simulink model "North_Country_Grid_2024a"  (R2024a)
settings: Solver=VariableStepAuto  StartTime=0.0  StopTime=10  RelTol=1e-3
PreLoadFcn:
  | Ts=50e-6;
InitFcn:
  | xInitial = WindFarmType4AverageModelInit;
  | Ts=50e-6;
undefined symbols (not defined in the file or in its folder): D1, D11, Delta, DiscIntNeverNeededParam, find_system, Fnom_I, Fnom_R, Idc_nom, lagging, level, pulse, test_alpha, Vdc_nom, VLL_nom_I, VLL_nom_R
libraries: spsSecondOrderFilterLib x47, powerlib_extras x38, simulink x34, spsThreePhaseVIMeasurementLib x30, spsFirstOrderFilterLib x29, simulink_extras x26, spsabctodq0Lib x25, spsThreePhaseTransformerTwoWindingsLib x19, spsThreePhaseBreakerLib x18, spsThreePhasePISectionLineLib x17, spsControlledVoltageSourceLib x15, spsOnDelayLib x12
(part 5 of 18)

== system North_Country_Grid_2024a/Noble Clinton (Type 4, 100.5 MW)/Wind Farm ==
  note: Turbine and Drive Train
  note: Control
  note: Output
  note: Inverter
      | Average Model
  note: DC-DC Boost Converter
      | Average Model
  "Wind (m/s) " : Inport
  Qref_pu : Inport  Port=2
  -> pu : Gain  Gain=1/(Pnom/(3*sqrt(2)/pi*Vnom_gen))  SaturateOnIntegerOverflow=on  OutDataTypeStr=Inherit: Same as input  ParamDataTypeStr=Inherit: Same as input
  Average Switch Voltage : Subsystem
  B_gen : spsThreePhaseVIMeasurementLib/Three-Phase V-I Measurement  VoltageMeasurement=phase-to-phase  SetLabelV=off  LabelV=Vabc  Vpu=on  VpuLL=off  CurrentMeasurement=yes  SetLabelI=off  LabelI=Iabc  Ipu=on  Pbase=Pnom  Vbase=Vnom_gen  OutputType=Complex  PhasorSimulation=off  PSBequivalent=0
  B_grid : spsThreePhaseVIMeasurementLib/Three-Phase V-I Measurement  VoltageMeasurement=phase-to-ground  SetLabelV=off  LabelV=Vabc  Vpu=on  VpuLL=off  CurrentMeasurement=yes  SetLabelI=off  LabelI=Iabc  Ipu=on  Pbase=Pnom  Vbase=Vnom  OutputType=Complex  PhasorSimulation=off  PSBequivalent=0
  B_grid_conv : spsThreePhaseVIMeasurementLib/Three-Phase V-I Measurement  VoltageMeasurement=phase-to-ground  SetLabelV=off  LabelV=Vabc  Vpu=on  VpuLL=off  CurrentMeasurement=no  SetLabelI=off  LabelI=Iabc  Ipu=on  Pbase=Pnom  Vbase=Vnom  OutputType=Complex  PhasorSimulation=off  PSBequivalent=0
  Bus Creator : BusCreator  Inputs=11
  Bus Selector : BusSelector  OutputSignals="Mechanical.Rotor speed  wm  (pu),Mechanical.Rotor mechanical angle  theta (deg)"
  "Choke " : spsThreePhaseSeriesRLCBranchLib/Three-Phase Series RLC Branch  LConnTagsString=A|B|C  RConnTagsString=A|B|C  BranchType=RL  Resistance=R_RL*Vnom^2/Pnom  Inductance=L_RL*Vnom^2/Pnom/(2*pi*Fnom)  Capacitance=[]  Measurements=None
  Control : Subsystem
  Drive Train : Subsystem  mask(Wind Turbine shaft){H_WT=H_WT, Ksh=Ksh, D_mutual=D_mutual, wbase=2*pi*Fnom/p, w_wt0=w_wt0, torque0=torque0, Ts=Ts}
      mask prompts: H_WT "Wind turbine inertia constant H (s):"; Ksh "Shaft spring constant (pu of nominal mechanical torque/rad):"; D_mutual "Shaft mutual damping (pu of nominal mechanical torque/pu dw):"; wbase "Shaft base speed (rad/s):"; w_wt0 "Turbine initial speed (pu of base speed):"; torque0 "Initial output torque (pu of nominal mechanical torque):"; Ts "Sample time (s):"
      mask help:
      | This block implements a wind turbine drive train model. All shaft parameters are referred to high-speed shaft (generator shaft).
      |
      | The first input is the wind turbine torque in per unit (pu) based on the nominal power of the turbine and the base speed of the generator. The second input is the generator speed in pu based on the base speed of the generator.
      |
      | The outputs are:
      | 1- the transmitted torque of the shaft in pu based on the nominal power of the turbine and the base speed of the generator.
      | 2- the wind turbine speed in pu of the base speed of the generator.
  Filter Q=50 : spsThreePhaseSeriesRLCLoadLib/Three-Phase Series RLC Load  LConnTagsString=A|B|C  Configuration=Y (grounded)  NominalVoltage=Vnom  Vabc=[1e3 1e3 1e3]  Vabcp=[1e3 1e3 1e3]  NominalFrequency=Fnom  UnbalancedPower=off  ActivePower=C_var_filter/Q_filter  InductivePower=0  CapacitivePower=C_var_filter  Pabc=[10e3 9e3 11e3]  QLabc=[100 90 110]  QCabc=[100 90 110]  Pabcp=[10e3 9e3 11e3]  QLabcp=[100 90 110]  QCabcp=[100 90 110]  Measurements=None  LoadType=constant Z
  IL : spsCurrentMeasurementLib/Current Measurement  PhasorSimulation=off  OutputType=Complex  PSBequivalent=0
  Inverter and DC-DC Converter Average Models : Subsystem
  Power base for the Generator : Gain  Gain=Pmec/Pnom  SaturateOnIntegerOverflow=on  OutDataTypeStr=Inherit: Same as input  ParamDataTypeStr=Inherit: Same as input
  Product : Product  RndMeth=Zero
  Series RLC Branch1 : spsSeriesRLCBranchLib/Series RLC Branch  LConnTagsString=__new0  RConnTagsString=__new0  BranchType=RL  Resistance=R_Boost  Inductance=L_Boost  SetiL0=off  InitialCurrent=0  Capacitance=1.0  Setx0=off  InitialVoltage=0  Measurements=Branch current
  Synchronous Machine pu Standard : spsSynchronousMachinepuStandardLib/Synchronous Machine pu Standard  PresetModel=No  MechanicalLoad=Mechanical power Pm  ShowDetailedParameters=on  RotorType=Salient-pole  Units=per unit standard parameters  MeasurementBus=off  NominalParameters="[ Pnom  Vnom_gen Fnom ]"  Reactances1=[ 1.81, 0.3, 0.23, 1.76, 0.65, 0.25, 0.15 ]  Reactances2="[ Xd, Xd1, Xd2, Xq,  Xq2,  Xl ]"  dAxisTimeConstants=Open-circuit  qAxisTimeConstants=Short-circuit  TimeConstants1="[ 4.4849  0.0681  0.1  ]"  TimeConstants2=[ 8.0, 0.03, 1.0, 0.07 ]  TimeConstants3="[  Tdo1  Tdo2  Tq2  ]"  TimeConstants4=[ 8.0, 0.03, 0.3371, 0.0295 ]  TimeConstants5=[ 1.01, 0.053, 0.1 ]  TimeConstants6=[ 1.3201, 0.023, 1.0, 0.07 ]  TimeConstants7="[  1.01  0.053  0.051266  ]"  TimeConstants8=[ 1.3201, 0.0231, 0.3371, 0.0295 ]  StatorResistance=Resistance  Mechanical=[ H F p]  PolePairs=1  InitialConditions=init  SetSaturation=off  Saturation=[0.6404,0.7127,0.8441,0.9214,0.9956,1.082,1.19,1.316,1.457;0.7,0.7698,0.8872,0.9466,0.9969,1.046,1.1,1.151,1.201]  LoadFlowParameters=[1,0,0,0,0]  TsPowergui=0  TsBlock=-1  IterativeModel=Trapezoidal non iterative  IterativeDiscreteModel=Trapezoidal non iterative  BusType=PV  Pref=0  Qref=0  Qmin=-inf  Qmax=inf  PLF=0  QLF=0
  Universal Bridge : spsUniversalBridgeLib/Universal Bridge  Arms=3  SnubberResistance=2*Ts_snub/(Pnom/(1000*2*pi*Fnom*Vnom_gen^2))  SnubberCapacitance=Pnom/(1000*2*pi*Fnom*Vnom_gen^2)  Device=Diodes  Ron=1e-6/Nb_wt  Lon=0  ForwardVoltages="[  0  0  ]"  ForwardVoltage=0  GTOparameters=[ 10e-6 , 20e-6 ]  IGBTparameters=[ 1e-6 , 2e-6 ]  Measurements=None  Measurements_2=None  converterType=Rectifier
  V_ab : spsControlledVoltageSourceLib/Controlled Voltage Source  Initialize=on  Source_Type=AC  Amplitude=0  Phase=0  Frequency=0  Measurements=None
  V_bc : spsControlledVoltageSourceLib/Controlled Voltage Source  Initialize=on  Source_Type=AC  Amplitude=0  Phase=0  Frequency=0  Measurements=None
  Wind Turbine : Subsystem  mask(Wind Turbine){Prated=Pmec, c1_c8=c1_c8, K1_K2=K1_K2, wind0=wind0, Ts=Ts}
      mask prompts: Prated "Nominal mechanical output power (W):"; c1_c8 "Coefficients [c1 ... c8]"; K1_K2 "Parameters [K1 K2]"; wind0 "Initial wind speed (m/s):"; Ts "Sample time (s):"
      mask help:
      | This block implements a generic wind turbine models.
      |
      | The first input is the turbine speed in per unit of the generator base speed. For a synchronous or asynchronous generator, the base speed is the synchronous speed. For a permanent-magnet generator, the base speed is defined as the speed producing nominal voltage at  no load. The second input is the blade pitch angle in degrees. The third input is the wind speed in m/s.
      |
      | The output is the torque applied to the drive train in per unit based on the nominal power of the turbine and the base speed of the generator.
      mask init:
      | c1 = c1_c8(1);
      | c2 = c1_c8(2);
      | c3 = c1_c8(3);
      | c4 = c1_c8(4);
      | c5 = c1_c8(5);
      | c6 = c1_c8(6);
      | c7 = c1_c8(7);;
      | c8 = c1_c8(8);
      | 
      | K1=K1_K2(1);
      | K2=K1_K2(2);
      settings: OpenFcn=power_openblockproxy();
      mask Display: disp('');
  deg->rd : Gain  Gain=pi/180  SaturateOnIntegerOverflow=on  OutDataTypeStr=Inherit: Same as input  ParamDataTypeStr=Inherit: Same as input
  A : PMIOPort  Tag=PMCPort  Side=Left
  B : PMIOPort  Tag=PMCPort  Port=2  Side=Left
  C : PMIOPort  Tag=PMCPort  Port=3  Side=Left
  m : Outport  VectorParamsAs1DForOutWhenUnconnected=off
  wires:
  Wind Turbine/1(Tt (pu)) -> Drive Train/1(T_wt (pu))
  [wr] -> Drive Train/2(Generator speed (pu))
  Drive Train/2(T_shaft (pu)) -> Power base for the Generator/1
  Power base for the Generator/1 -> [Tm]
  "Wind (m/s) "/1 -> Wind Turbine/3(Wind speed (m/s))
  Drive Train/1(W_wt (pu)) -> Wind Turbine/1(W_wt (pu))
  [Pitch] -> Wind Turbine/2(Pitch angle (deg))
  Bus Selector/2 -> deg->rd/1  "<Rotor mechanical angle  theta (deg)>"
  deg->rd/1 -> [angle_rotor]
  Bus Selector/1 -> [wr]  "<Rotor speed  wm  (pu)>"
  [wr] -> Product/1
  Synchronous Machine pu Standard/1 -> Bus Selector/1
  B_grid_conv/1 -> [Vabc_grid_conv]
  [Vabc_LL_stator] -> Bus Creator/1  "Vabc_stator_pu"
  [Iabc_stator] -> Bus Creator/2  "Iabc_stator_pu"
  [Vabc_grid] -> Bus Creator/3  "Vabc_grid_pu"
  Bus Creator/1 -> m/1
  [Vabc_grid_conv] -> Bus Creator/4  "Vabc_grid_conv_pu"
  [Iabc_grid_conv] -> Bus Creator/5  "Iabc_grid_conv_pu"
  [Vf] -> Bus Creator/6  "Vfield_pu"
  [wr] -> Bus Creator/7  "wr_pu"
  [Pm_gen] -> Bus Creator/8  "Pm_gen_pu"
  [Pitch] -> Bus Creator/9  "Pitch_deg"
  [Vdc] -> Bus Creator/10  "Vdc_V"
  [Tm] -> Product/2
  Product/1 -> Synchronous Machine pu Standard/1, [Pm_gen]
  [Iabc_grid_conv] -> Inverter and DC-DC Converter Average Models/2(Iabc_grid_conv)
  Inverter and DC-DC Converter Average Models/3(Vswitch (V)) -> Average Switch Voltage/1(Vswitch)
  IL/1 -> -> pu/1
  [IL] -> Inverter and DC-DC Converter Average Models/1(IL)
  B_grid/1 -> [Vabc_grid]
  B_grid/2 -> [Iabc_grid_conv]
  B_gen/1 -> [Vabc_LL_stator]
  B_gen/2 -> [Iabc_stator]
  [Vabc_grid] -> Control/1(Vabc_grid)
  [Iabc_grid_conv] -> Control/2(Iabc_grid_conv)
  [Vabc_LL_stator] -> Control/3(Vabc_LL_stator)
  [Iabc_stator] -> Control/4(Iabc_stator)
  [Vdc] -> Control/6(Vdc)
  Qref_pu/1 -> Control/7(Qref)
  [angle_rotor] -> Control/8(angle_rotor)
  [wr] -> Control/9(wr)
  Control/1(Uctrl_inverter) -> Inverter and DC-DC Converter Average Models/3(Uctrl_inverter)
  Control/2(Duty_Cycle) -> Inverter and DC-DC Converter Average Models/4(Duty_Cycle)  "Duty_cycle"
  Control/3(Pitch_angle) -> [Pitch]
  Control/4(Vf) -> [Vf]
  Inverter and DC-DC Converter Average Models/4(Vdc (V)) -> [Vdc]
  [Vf] -> Synchronous Machine pu Standard/2
  Inverter and DC-DC Converter Average Models/1(Vab (V)) -> V_ab/1
  Inverter and DC-DC Converter Average Models/2(Vbc (V)) -> V_bc/1
  Control/5(PQ_pu) -> [PQ_pu]
  [PQ_pu] -> Bus Creator/11  "PQ_pu"
  [IL] -> Control/5(IL)
  -> pu/1 -> [IL]
  connections:
  B_gen/RConn1 -- Synchronous Machine pu Standard/RConn1
  B_gen/RConn2 -- Synchronous Machine pu Standard/RConn2
  B_gen/RConn3 -- Synchronous Machine pu Standard/RConn3
  B_grid/RConn1 -- "Choke "/LConn1
  B_grid/RConn2 -- "Choke "/LConn2
  B_grid/RConn3 -- "Choke "/LConn3
  B_grid/LConn1 -- A/RConn1 -- Filter Q=50/LConn1
  B/RConn1 -- B_grid/LConn2 -- Filter Q=50/LConn2
  C/RConn1 -- B_grid/LConn3 -- Filter Q=50/LConn3
  "Choke "/RConn1 -- B_grid_conv/LConn1
  "Choke "/RConn2 -- B_grid_conv/LConn2
  "Choke "/RConn3 -- B_grid_conv/LConn3
  Series RLC Branch1/LConn1 -- Universal Bridge/RConn1
  Average Switch Voltage/LConn1 -- Universal Bridge/RConn2
  V_ab/RConn1 -- B_grid_conv/RConn1
  B_grid_conv/RConn3 -- V_bc/LConn1
  V_bc/RConn1 -- V_ab/LConn1 -- B_grid_conv/RConn2
  Universal Bridge/LConn1 -- B_gen/LConn1
  Universal Bridge/LConn2 -- B_gen/LConn2
  Universal Bridge/LConn3 -- B_gen/LConn3
  Series RLC Branch1/RConn1 -- IL/LConn1
  Average Switch Voltage/RConn1 -- IL/RConn1

== system North_Country_Grid_2024a/Noble Ellenburg (Type 4, 81 MW)/Wind Farm ==
  note: Turbine and Drive Train
  note: Control
  note: Output
  note: Inverter
      | Average Model
  note: DC-DC Boost Converter
      | Average Model
  "Wind (m/s) " : Inport
  Qref_pu : Inport  Port=2
  -> pu : Gain  Gain=1/(Pnom/(3*sqrt(2)/pi*Vnom_gen))  SaturateOnIntegerOverflow=on  OutDataTypeStr=Inherit: Same as input  ParamDataTypeStr=Inherit: Same as input
  Average Switch Voltage : Subsystem
  B_gen : spsThreePhaseVIMeasurementLib/Three-Phase V-I Measurement  VoltageMeasurement=phase-to-phase  SetLabelV=off  LabelV=Vabc  Vpu=on  VpuLL=off  CurrentMeasurement=yes  SetLabelI=off  LabelI=Iabc  Ipu=on  Pbase=Pnom  Vbase=Vnom_gen  OutputType=Complex  PhasorSimulation=off  PSBequivalent=0
  B_grid : spsThreePhaseVIMeasurementLib/Three-Phase V-I Measurement  VoltageMeasurement=phase-to-ground  SetLabelV=off  LabelV=Vabc  Vpu=on  VpuLL=off  CurrentMeasurement=yes  SetLabelI=off  LabelI=Iabc  Ipu=on  Pbase=Pnom  Vbase=Vnom  OutputType=Complex  PhasorSimulation=off  PSBequivalent=0
  B_grid_conv : spsThreePhaseVIMeasurementLib/Three-Phase V-I Measurement  VoltageMeasurement=phase-to-ground  SetLabelV=off  LabelV=Vabc  Vpu=on  VpuLL=off  CurrentMeasurement=no  SetLabelI=off  LabelI=Iabc  Ipu=on  Pbase=Pnom  Vbase=Vnom  OutputType=Complex  PhasorSimulation=off  PSBequivalent=0
  Bus Creator : BusCreator  Inputs=11
  Bus Selector : BusSelector  OutputSignals="Mechanical.Rotor speed  wm  (pu),Mechanical.Rotor mechanical angle  theta (deg)"
  "Choke " : spsThreePhaseSeriesRLCBranchLib/Three-Phase Series RLC Branch  LConnTagsString=A|B|C  RConnTagsString=A|B|C  BranchType=RL  Resistance=R_RL*Vnom^2/Pnom  Inductance=L_RL*Vnom^2/Pnom/(2*pi*Fnom)  Capacitance=[]  Measurements=None
  Control : Subsystem
  Drive Train : Subsystem  mask(Wind Turbine shaft){H_WT=H_WT, Ksh=Ksh, D_mutual=D_mutual, wbase=2*pi*Fnom/p, w_wt0=w_wt0, torque0=torque0, Ts=Ts}
      mask prompts: H_WT "Wind turbine inertia constant H (s):"; Ksh "Shaft spring constant (pu of nominal mechanical torque/rad):"; D_mutual "Shaft mutual damping (pu of nominal mechanical torque/pu dw):"; wbase "Shaft base speed (rad/s):"; w_wt0 "Turbine initial speed (pu of base speed):"; torque0 "Initial output torque (pu of nominal mechanical torque):"; Ts "Sample time (s):"
      mask help:
      | This block implements a wind turbine drive train model. All shaft parameters are referred to high-speed shaft (generator shaft).
      |
      | The first input is the wind turbine torque in per unit (pu) based on the nominal power of the turbine and the base speed of the generator. The second input is the generator speed in pu based on the base speed of the generator.
      |
      | The outputs are:
      | 1- the transmitted torque of the shaft in pu based on the nominal power of the turbine and the base speed of the generator.
      | 2- the wind turbine speed in pu of the base speed of the generator.
  Filter Q=50 : spsThreePhaseSeriesRLCLoadLib/Three-Phase Series RLC Load  LConnTagsString=A|B|C  Configuration=Y (grounded)  NominalVoltage=Vnom  Vabc=[1e3 1e3 1e3]  Vabcp=[1e3 1e3 1e3]  NominalFrequency=Fnom  UnbalancedPower=off  ActivePower=C_var_filter/Q_filter  InductivePower=0  CapacitivePower=C_var_filter  Pabc=[10e3 9e3 11e3]  QLabc=[100 90 110]  QCabc=[100 90 110]  Pabcp=[10e3 9e3 11e3]  QLabcp=[100 90 110]  QCabcp=[100 90 110]  Measurements=None  LoadType=constant Z
  IL : spsCurrentMeasurementLib/Current Measurement  PhasorSimulation=off  OutputType=Complex  PSBequivalent=0
  Inverter and DC-DC Converter Average Models : Subsystem
  Power base for the Generator : Gain  Gain=Pmec/Pnom  SaturateOnIntegerOverflow=on  OutDataTypeStr=Inherit: Same as input  ParamDataTypeStr=Inherit: Same as input
  Product : Product  RndMeth=Zero
  Series RLC Branch1 : spsSeriesRLCBranchLib/Series RLC Branch  LConnTagsString=__new0  RConnTagsString=__new0  BranchType=RL  Resistance=R_Boost  Inductance=L_Boost  SetiL0=off  InitialCurrent=0  Capacitance=1.0  Setx0=off  InitialVoltage=0  Measurements=Branch current
  Synchronous Machine pu Standard : spsSynchronousMachinepuStandardLib/Synchronous Machine pu Standard  PresetModel=No  MechanicalLoad=Mechanical power Pm  ShowDetailedParameters=on  RotorType=Salient-pole  Units=per unit standard parameters  MeasurementBus=off  NominalParameters="[ Pnom  Vnom_gen Fnom ]"  Reactances1=[ 1.81, 0.3, 0.23, 1.76, 0.65, 0.25, 0.15 ]  Reactances2="[ Xd, Xd1, Xd2, Xq,  Xq2,  Xl ]"  dAxisTimeConstants=Open-circuit  qAxisTimeConstants=Short-circuit  TimeConstants1="[ 4.4849  0.0681  0.1  ]"  TimeConstants2=[ 8.0, 0.03, 1.0, 0.07 ]  TimeConstants3="[  Tdo1  Tdo2  Tq2  ]"  TimeConstants4=[ 8.0, 0.03, 0.3371, 0.0295 ]  TimeConstants5=[ 1.01, 0.053, 0.1 ]  TimeConstants6=[ 1.3201, 0.023, 1.0, 0.07 ]  TimeConstants7="[  1.01  0.053  0.051266  ]"  TimeConstants8=[ 1.3201, 0.0231, 0.3371, 0.0295 ]  StatorResistance=Resistance  Mechanical=[ H F p]  PolePairs=1  InitialConditions=init  SetSaturation=off  Saturation=[0.6404,0.7127,0.8441,0.9214,0.9956,1.082,1.19,1.316,1.457;0.7,0.7698,0.8872,0.9466,0.9969,1.046,1.1,1.151,1.201]  LoadFlowParameters=[1 0 0 0 0]  TsPowergui=0  TsBlock=-1  IterativeModel=Trapezoidal non iterative  IterativeDiscreteModel=Trapezoidal non iterative  BusType=PV  Pref=0  Qref=0  Qmin=-inf  Qmax=inf  PLF=0  QLF=0
  Universal Bridge : spsUniversalBridgeLib/Universal Bridge  Arms=3  SnubberResistance=2*Ts_snub/(Pnom/(1000*2*pi*Fnom*Vnom_gen^2))  SnubberCapacitance=Pnom/(1000*2*pi*Fnom*Vnom_gen^2)  Device=Diodes  Ron=1e-6/Nb_wt  Lon=0  ForwardVoltages="[  0  0  ]"  ForwardVoltage=0  GTOparameters=[ 10e-6 , 20e-6 ]  IGBTparameters=[ 1e-6 , 2e-6 ]  Measurements=None  Measurements_2=None  converterType=Rectifier
  V_ab : spsControlledVoltageSourceLib/Controlled Voltage Source  Initialize=on  Source_Type=AC  Amplitude=0  Phase=0  Frequency=0  Measurements=None
  V_bc : spsControlledVoltageSourceLib/Controlled Voltage Source  Initialize=on  Source_Type=AC  Amplitude=0  Phase=0  Frequency=0  Measurements=None
  Wind Turbine : Subsystem  mask(Wind Turbine){Prated=Pmec, c1_c8=c1_c8, K1_K2=K1_K2, wind0=wind0, Ts=Ts}
      mask prompts: Prated "Nominal mechanical output power (W):"; c1_c8 "Coefficients [c1 ... c8]"; K1_K2 "Parameters [K1 K2]"; wind0 "Initial wind speed (m/s):"; Ts "Sample time (s):"
      mask help:
      | This block implements a generic wind turbine models.
      |
      | The first input is the turbine speed in per unit of the generator base speed. For a synchronous or asynchronous generator, the base speed is the synchronous speed. For a permanent-magnet generator, the base speed is defined as the speed producing nominal voltage at  no load. The second input is the blade pitch angle in degrees. The third input is the wind speed in m/s.
      |
      | The output is the torque applied to the drive train in per unit based on the nominal power of the turbine and the base speed of the generator.
      mask init:
      | c1 = c1_c8(1);
      | c2 = c1_c8(2);
      | c3 = c1_c8(3);
      | c4 = c1_c8(4);
      | c5 = c1_c8(5);
      | c6 = c1_c8(6);
      | c7 = c1_c8(7);;
      | c8 = c1_c8(8);
      | 
      | K1=K1_K2(1);
      | K2=K1_K2(2);
      settings: OpenFcn=power_openblockproxy();
      mask Display: disp('');
  deg->rd : Gain  Gain=pi/180  SaturateOnIntegerOverflow=on  OutDataTypeStr=Inherit: Same as input  ParamDataTypeStr=Inherit: Same as input
  A : PMIOPort  Tag=PMCPort  Side=Left
  B : PMIOPort  Tag=PMCPort  Port=2  Side=Left
  C : PMIOPort  Tag=PMCPort  Port=3  Side=Left
  m : Outport  VectorParamsAs1DForOutWhenUnconnected=off
  wires:
  Wind Turbine/1(Tt (pu)) -> Drive Train/1(T_wt (pu))
  [wr] -> Drive Train/2(Generator speed (pu))
  Drive Train/2(T_shaft (pu)) -> Power base for the Generator/1
  Power base for the Generator/1 -> [Tm]
  "Wind (m/s) "/1 -> Wind Turbine/3(Wind speed (m/s))
  Drive Train/1(W_wt (pu)) -> Wind Turbine/1(W_wt (pu))
  [Pitch] -> Wind Turbine/2(Pitch angle (deg))
  Bus Selector/2 -> deg->rd/1  "<Rotor mechanical angle  theta (deg)>"
  deg->rd/1 -> [angle_rotor]
  Bus Selector/1 -> [wr]  "<Rotor speed  wm  (pu)>"
  [wr] -> Product/1
  Synchronous Machine pu Standard/1 -> Bus Selector/1
  B_grid_conv/1 -> [Vabc_grid_conv]
  [Vabc_LL_stator] -> Bus Creator/1  "Vabc_stator_pu"
  [Iabc_stator] -> Bus Creator/2  "Iabc_stator_pu"
  [Vabc_grid] -> Bus Creator/3  "Vabc_grid_pu"
  Bus Creator/1 -> m/1
  [Vabc_grid_conv] -> Bus Creator/4  "Vabc_grid_conv_pu"
  [Iabc_grid_conv] -> Bus Creator/5  "Iabc_grid_conv_pu"
  [Vf] -> Bus Creator/6  "Vfield_pu"
  [wr] -> Bus Creator/7  "wr_pu"
  [Pm_gen] -> Bus Creator/8  "Pm_gen_pu"
  [Pitch] -> Bus Creator/9  "Pitch_deg"
  [Vdc] -> Bus Creator/10  "Vdc_V"
  [Tm] -> Product/2
  Product/1 -> Synchronous Machine pu Standard/1, [Pm_gen]
  [Iabc_grid_conv] -> Inverter and DC-DC Converter Average Models/2(Iabc_grid_conv)
  Inverter and DC-DC Converter Average Models/3(Vswitch (V)) -> Average Switch Voltage/1(Vswitch)
  IL/1 -> -> pu/1
  [IL] -> Inverter and DC-DC Converter Average Models/1(IL)
  B_grid/1 -> [Vabc_grid]
  B_grid/2 -> [Iabc_grid_conv]
  B_gen/1 -> [Vabc_LL_stator]
  B_gen/2 -> [Iabc_stator]
  [Vabc_grid] -> Control/1(Vabc_grid)
  [Iabc_grid_conv] -> Control/2(Iabc_grid_conv)
  [Vabc_LL_stator] -> Control/3(Vabc_LL_stator)
  [Iabc_stator] -> Control/4(Iabc_stator)
  [Vdc] -> Control/6(Vdc)
  Qref_pu/1 -> Control/7(Qref)
  [angle_rotor] -> Control/8(angle_rotor)
  [wr] -> Control/9(wr)
  Control/1(Uctrl_inverter) -> Inverter and DC-DC Converter Average Models/3(Uctrl_inverter)
  Control/2(Duty_Cycle) -> Inverter and DC-DC Converter Average Models/4(Duty_Cycle)  "Duty_cycle"
  Control/3(Pitch_angle) -> [Pitch]
  Control/4(Vf) -> [Vf]
  Inverter and DC-DC Converter Average Models/4(Vdc (V)) -> [Vdc]
  [Vf] -> Synchronous Machine pu Standard/2
  Inverter and DC-DC Converter Average Models/1(Vab (V)) -> V_ab/1
  Inverter and DC-DC Converter Average Models/2(Vbc (V)) -> V_bc/1
  Control/5(PQ_pu) -> [PQ_pu]
  [PQ_pu] -> Bus Creator/11  "PQ_pu"
  [IL] -> Control/5(IL)
  -> pu/1 -> [IL]
  connections:
  B_gen/RConn1 -- Synchronous Machine pu Standard/RConn1
  B_gen/RConn2 -- Synchronous Machine pu Standard/RConn2
  B_gen/RConn3 -- Synchronous Machine pu Standard/RConn3
  B_grid/RConn1 -- "Choke "/LConn1
  B_grid/RConn2 -- "Choke "/LConn2
  B_grid/RConn3 -- "Choke "/LConn3
  B_grid/LConn1 -- A/RConn1 -- Filter Q=50/LConn1
  B/RConn1 -- B_grid/LConn2 -- Filter Q=50/LConn2
  C/RConn1 -- B_grid/LConn3 -- Filter Q=50/LConn3
  "Choke "/RConn1 -- B_grid_conv/LConn1
  "Choke "/RConn2 -- B_grid_conv/LConn2
  "Choke "/RConn3 -- B_grid_conv/LConn3
  Series RLC Branch1/LConn1 -- Universal Bridge/RConn1
  Average Switch Voltage/LConn1 -- Universal Bridge/RConn2
  V_ab/RConn1 -- B_grid_conv/RConn1
  B_grid_conv/RConn3 -- V_bc/LConn1
  V_bc/RConn1 -- V_ab/LConn1 -- B_grid_conv/RConn2
  Universal Bridge/LConn1 -- B_gen/LConn1
  Universal Bridge/LConn2 -- B_gen/LConn2
  Universal Bridge/LConn3 -- B_gen/LConn3
  Series RLC Branch1/RConn1 -- IL/LConn1
  Average Switch Voltage/RConn1 -- IL/RConn1

== system North_Country_Grid_2024a/Chateauguay HVDC Back-to-Back Converter/Inverter/Inverter ==
  Py : Inport
  Pd : Inport  Port=2
  Bridge D : spsUniversalBridgeLib/Universal Bridge  Arms=3  SnubberResistance=2000  SnubberCapacitance=0.1e-6  Device=Thyristors  Ron=1e-3  Lon=0  ForwardVoltages="[  0.8  0.8  ]"  ForwardVoltage=0  GTOparameters=[ 10e-6 , 20e-6 ]  IGBTparameters=[ 1e-6 , 2e-6 ]  Measurements=Device currents  Measurements_2=None  converterType=Rectifier
      settings: AttributesFormatString=\n
  Bridge Y : spsUniversalBridgeLib/Universal Bridge  Arms=3  SnubberResistance=2000  SnubberCapacitance=0.1e-6  Device=Thyristors  Ron=1e-3  Lon=0  ForwardVoltages="[  0.8  0.8  ]"  ForwardVoltage=0  GTOparameters=[ 10e-6 , 20e-6 ]  IGBTparameters=[ 1e-6 , 2e-6 ]  Measurements=All voltages and currents  Measurements_2=None  converterType=Rectifier
      settings: AttributesFormatString=\n
  Ay : PMIOPort  Side=Left
  By : PMIOPort  Port=2  Side=Left
  Cy : PMIOPort  Port=3  Side=Left
  Ad : PMIOPort  Port=4  Side=Left
  Bd : PMIOPort  Port=5  Side=Left
  Cd : PMIOPort  Port=6  Side=Left
  pos : PMIOPort  Port=7  Side=Right
  neg : PMIOPort  Port=8  Side=Right
  wires:
  Py/1 -> Bridge Y/1
  Pd/1 -> Bridge D/1
  connections:
  Bridge D/RConn1 -- neg/RConn1
  Bridge Y/RConn2 -- pos/RConn1
  Bridge D/RConn2 -- Bridge Y/RConn1
  Ay/RConn1 -- Bridge Y/LConn1
  By/RConn1 -- Bridge Y/LConn2
  Cy/RConn1 -- Bridge Y/LConn3
  Ad/RConn1 -- Bridge D/LConn1
  Bd/RConn1 -- Bridge D/LConn2
  Cd/RConn1 -- Bridge D/LConn3

== system North_Country_Grid_2024a/Chateauguay HVDC Back-to-Back Converter/Inverter Control and Protection/12-pulse Firing Control ==
  alpha_ord (deg) : Inport
  Vabc (pu) : Inport  Port=2
  Block : Inport  Port=3
  PLL (3ph) : spsPLL3phLib/PLL (3ph)  Fmin=0.75 * PLL_f0  Par_Init="[PLL_ph  PLL_f0]"  ParK="[PLL_Kp  PLL_Ki  0]"  TcD=1e-4  MaxRateChangeFreq=12  FilterCutOffFreq=25  Ts=Ts  AGC=off
  "Pulse Generator (Thyristor, 12-Pulse)" : spsPulseGeneratorThyristor12PulseLib/Pulse Generator (Thyristor, 12-Pulse)  GenType=12-pulse  Delta=D1 (lagging)  pwidth=Pw  Double_Pulse=off  Ts=Ts
  PulsesY : Outport  VectorParamsAs1DForOutWhenUnconnected=off
  PulsesD : Outport  Port=2  VectorParamsAs1DForOutWhenUnconnected=off
  Freq : Outport  Port=3  VectorParamsAs1DForOutWhenUnconnected=off
  wires:
  Vabc (pu)/1 -> PLL (3ph)/1
  PLL (3ph)/2 -> "Pulse Generator (Thyristor, 12-Pulse)"/2
  alpha_ord (deg)/1 -> "Pulse Generator (Thyristor, 12-Pulse)"/1
  "Pulse Generator (Thyristor, 12-Pulse)"/1 -> PulsesY/1
  "Pulse Generator (Thyristor, 12-Pulse)"/2 -> PulsesD/1
  PLL (3ph)/1 -> Freq/1
  Block/1 -> "Pulse Generator (Thyristor, 12-Pulse)"/3

== system North_Country_Grid_2024a/Chateauguay HVDC Back-to-Back Converter/Inverter Control and Protection/Gamma Measurement ==
  Vabc : Inport
  I_th(1-6)_Y : Inport  Port=2
  I_th(1-6)_D : Inport  Port=3
  Freq : Inport  Port=4
  PulsesY : Inport  Port=5
  PulsesD : Inport  Port=6
  A--> pu : Gain  Gain=1/Idc_nom  SaturateOnIntegerOverflow=on  OutDataTypeStr=Inherit: Same as input  ParamDataTypeStr=Inherit: Same as input
  "A--> pu " : Gain  Gain=1/Idc_nom  SaturateOnIntegerOverflow=on  OutDataTypeStr=Inherit: Same as input  ParamDataTypeStr=Inherit: Same as input
  Gamma Measurement (D1 bridge) : Subsystem  DialogController=POWERSYS.PowerSysDialog  mask(Discrete Gamma Measurement (6-pulse converter)){transfo_type=Yg / D1(lag), f0=Fnom_I, Ith_min=0.001, Interpolation=on, V_tol=0.01, Ts=Ts}
      mask prompts: transfo_type "Transformer connection:"; f0 "Base frequency (Hz):"; Ith_min "Current threshold for thyristor zero-current detection (pu or A):"; Interpolation "Use interpolation"; V_tol "Voltage threshold for linear interpolation  (pu or V):"; Ts "Sample time (s):"
      mask help:
      | This block measures the extinction angle Gamma of a 6-pulse thyristor converter.
      |
      | Press Help for details.
      mask init:
      | powericon('psbcallbacks',gcb,'Discrete Gamma Measurement');
      | power_initmask();
      | if strcmp(Interpolation,'on')
      |     InterpolationOn=1;
      | else
      |     InterpolationOn=0;
      | end
      mask Help:
      | This block measures the extinction angle Gamma for each of the 6 thyristors
      | of a 6-pulse thyristor converter.
      | 
      | Gamma is the time expressed in degrees from the thyristor normal current
      | extinction to the time when the thyristor commutation voltage Vak becomes
      | positive. If interpolation is activated, Gamma is evaluated more precisely
      | by predicting the "exact" zero crossing instant of commutation voltage.
      | Interpolation is applied only if the voltage variation between the two
      | voltage samples on each side of zero-crossing exceeds the value specified
      | in the "Voltage threshold for interpolation" parameter (recommended value
      | 1% of nominal voltage).
      | 
      | The system frequency (input 3) is used to convert time values in electrical
      |  degrees. The current extinction time is determined from the "Current
      | threshold" parameter (recommended value 0.1% of nominal current). Valve
      | gate pulses (input 4) are used to discriminate between a current extinction
      |  during normal commutation sequence (valve gate pulse no longer present)
      | and premature extinction due to current discontinuity when DC current
      | reference Id_ref is low, (typically Id_ref<0.1 pu). If gate pulses are not
      | connected to input 4, Gamma measurement will stay correct as long as there
      | is no discontinuity in valve current pulses.
      | 
      | The 6 Gamma angles are determined using the 6 thyristor currents (input 1)
      | and the 6 commutation voltages derived from the three phase-to-ground AC
      | voltages measured at the primary of the converter transformer (input 2).
      | The secondary winding connection of the converter transformer (Y or Delta)
      | is selectable from the "Transformer connection" parameter. This information
      |  is important to derive the correct commutation voltage, for the outgoing
      | valve, from the primary voltages.
      | 
      | Output 1 = minimum value of the 6 Gamma angles over a rolling window of 6
      | consecutive extinctions; Output 2= mean value of the 6 Gamma angles; Output
      |  3 = vector of 6 commutation voltages used in the determination of Gamma,
      | assuming a 1:1 converter transformer ratio; Output 4= scalar output of the
      | six gamma angles.
      mask TypeOptions transfo_type: Yg / Y | Yg / D1(lag) | Yg / D11(lead)
      mask Callback Interpolation: powericon('psbcallbacks',gcb,'Discrete Gamma Measurement');
      mask Display: disp('\n\n\n')
  Gamma Measurement (Y bridge) : Subsystem  DialogController=POWERSYS.PowerSysDialog  mask(Discrete Gamma Measurement (6-pulse converter)){transfo_type=Yg / Y, f0=Fnom_I, Ith_min=0.001, Interpolation=on, V_tol=0.01, Ts=Ts}
      mask prompts: transfo_type "Transformer connection:"; f0 "Base frequency (Hz):"; Ith_min "Current threshold for thyristor zero-current detection (pu or A):"; Interpolation "Use interpolation"; V_tol "Voltage threshold for linear interpolation  (pu or V):"; Ts "Sample time (s):"
      mask help:
      | This block measures the extinction angle Gamma of a 6-pulse thyristor converter.
      |
      | Press Help for details.
      mask init:
      | powericon('psbcallbacks',gcb,'Discrete Gamma Measurement');
      | power_initmask();
      | if strcmp(Interpolation,'on')
      |     InterpolationOn=1;
      | else
      |     InterpolationOn=0;
      | end
      mask Help:
      | This block measures the extinction angle Gamma for each of the 6 thyristors
      | of a 6-pulse thyristor converter.
      | 
      | Gamma is the time expressed in degrees from the thyristor normal current
      | extinction to the time when the thyristor commutation voltage Vak becomes
      | positive. If interpolation is activated, Gamma is evaluated more precisely
      | by predicting the "exact" zero crossing instant of commutation voltage.
      | Interpolation is applied only if the voltage variation between the two
      | voltage samples on each side of zero-crossing exceeds the value specified
      | in the "Voltage threshold for interpolation" parameter (recommended value
      | 1% of nominal voltage).
      | 
      | The system frequency (input 3) is used to convert time values in electrical
      |  degrees. The current extinction time is determined from the "Current
      | threshold" parameter (recommended value 0.1% of nominal current). Valve
      | gate pulses (input 4) are used to discriminate between a current extinction
      |  during normal commutation sequence (valve gate pulse no longer present)
      | and premature extinction due to current discontinuity when DC current
      | reference Id_ref is low, (typically Id_ref<0.1 pu). If gate pulses are not
      | connected to input 4, Gamma measurement will stay correct as long as there
      | is no discontinuity in valve current pulses.
      | 
      | The 6 Gamma angles are determined using the 6 thyristor currents (input 1)
      | and the 6 commutation voltages derived from the three phase-to-ground AC
      | voltages measured at the primary of the converter transformer (input 2).
      | The secondary winding connection of the converter transformer (Y or Delta)
      | is selectable from the "Transformer connection" parameter. This information
      |  is important to derive the correct commutation voltage, for the outgoing
      | valve, from the primary voltages.
      | 
      | Output 1 = minimum value of the 6 Gamma angles over a rolling window of 6
      | consecutive extinctions; Output 2= mean value of the 6 Gamma angles; Output
      |  3 = vector of 6 commutation voltages used in the determination of Gamma,
      | assuming a 1:1 converter transformer ratio; Output 4= scalar output of the
      | six gamma angles.
      mask TypeOptions transfo_type: Yg / Y | Yg / D1(lag) | Yg / D11(lead)
      mask Callback Interpolation: powericon('psbcallbacks',gcb,'Discrete Gamma Measurement');
      mask Display: disp('\n\n\n')
  MinMax1 : MinMax  Inputs=2  InputSameDT=on  SaturateOnIntegerOverflow=on
  Selector : Selector  InputPortWidth=6  IndexOptions=Index vector (dialog)  Indices=1  OutputSizes=1
  Selector1 : Selector  InputPortWidth=6  IndexOptions=Index vector (dialog)  Indices=1  OutputSizes=1
  Sum1 : Sum  InputSameDT=on  SaturateOnIntegerOverflow=on  OutDataTypeStr=Inherit: Same as first input
  Terminator1 : Terminator
  Terminator2 : Terminator
  Terminator3 : Terminator
  k : Gain  Gain=0.5  SaturateOnIntegerOverflow=on  OutDataTypeStr=Inherit: Same as input  ParamDataTypeStr=Inherit: Same as input
  gamma_min : Outport  VectorParamsAs1DForOutWhenUnconnected=off
  gamma_mean : Outport  Port=2  VectorParamsAs1DForOutWhenUnconnected=off
  tag scope: ISw1Y_pu=global, Ucom1Y_pu=global
  wires:
  I_th(1-6)_Y/1 -> A--> pu/1
  A--> pu/1 -> Gamma Measurement (Y bridge)/1(I_th(1-6)), Selector1/1
  Vabc/1 -> Gamma Measurement (D1 bridge)/2(Uabc), Gamma Measurement (Y bridge)/2(Uabc)
  Gamma Measurement (Y bridge)/1(gamma_min (deg)) -> MinMax1/1  "gamma min Y"
  Gamma Measurement (Y bridge)/3(Ucom(1-6)) -> Selector/1
  Gamma Measurement (Y bridge)/2(gamma_mean (deg)) -> Sum1/1
  I_th(1-6)_D/1 -> "A--> pu "/1
  "A--> pu "/1 -> Gamma Measurement (D1 bridge)/1(I_th(1-6))
  Gamma Measurement (D1 bridge)/3(Ucom(1-6)) -> Terminator2/1
  Gamma Measurement (D1 bridge)/2(gamma_mean (deg)) -> Sum1/2
  Gamma Measurement (D1 bridge)/1(gamma_min (deg)) -> MinMax1/2  "gamma min D"
  MinMax1/1 -> gamma_min/1
  Sum1/1 -> k/1
  k/1 -> gamma_mean/1
  Selector/1 -> [Ucom1Y_pu]
  Selector1/1 -> [ISw1Y_pu]
  Freq/1 -> Gamma Measurement (D1 bridge)/3(Freq), Gamma Measurement (Y bridge)/3(Freq)
  Gamma Measurement (D1 bridge)/4(gamma (deg)) -> Terminator1/1
  Gamma Measurement (Y bridge)/4(gamma (deg)) -> Terminator3/1
  PulsesY/1 -> Gamma Measurement (Y bridge)/4(Pulses(1-6))
  PulsesD/1 -> Gamma Measurement (D1 bridge)/4(Pulses(1-6))

== system North_Country_Grid_2024a/Chateauguay HVDC Back-to-Back Converter/Inverter Control and Protection/Inverter Pole Control (Current//Voltage//Gamma) ==
  note: DISCRETE HVDC CONTROLLER
  note: Silvano Casoria
      | Power System Simulation Laboratory
      |  IREQ, Hydro-Quebec
  note: f0 =15 Hz
  VdL (pu) : Inport
  Id (pu) : Inport  Port=2
  Id_ref (pu) : Inport  Port=3
  Vd_ref (pu) : Inport  Port=4
  Block : Inport  Port=5
  Forced_alpha : Inport  Port=6
  gamma_meas (deg) : Inport  Port=7
  gamma_ref (deg) : Inport  Port=8
  D_alpha (deg) : Inport  Port=9
  Alpha Control : Subsystem
  Constant1 : Constant  Value=0
  Constant10 : Constant  Value=Mode
  Constant2 : Constant  Value=Inverter
  Constant4 : Constant  Value=Id_marg
  Constant5 : Constant  Value=Max_lin
  Constant6 : Constant  Value=Min_lin
  Constant8 : Constant  Value=180
  Constant9 : Constant  Value=180
  "Control Mode " : Subsystem
  Current Error : Sum  Inputs=++-  InputSameDT=on  SaturateOnIntegerOverflow=on  OutDataTypeStr=Inherit: Same as first input
  Current Regulator : Subsystem  TreatAsAtomicUnit=on
  First-Order Filter (T = T_I) : spsFirstOrderFilterLib/First-Order Filter  FilterType=Lowpass  Tc=T_I  Ts=Ts  Initialize=off  Vac_Init=[0, 0, 60]  Vdc_Init=0  PlotResponse=off  FreqRange="[0,  200,  1]"
  GR : Fcn  Expr=(u[1] == 2) || (u[1] == 4)
  Gamma Error : Subsystem  TreatAsAtomicUnit=on
  Gamma Regulator : Subsystem  TreatAsAtomicUnit=on
  Min=0 Max = 10 : Saturate  UpperLimit=10  LowerLimit=0
  MinMax : MinMax  Inputs=3  InputSameDT=on  SaturateOnIntegerOverflow=on
  Second-Order Filter (fn= f0_V) : spsSecondOrderFilterLib/Second-Order Filter  FilterType=Lowpass  Fo=f0_V  Zeta=Z_V  Ts=Ts  Initialize=off  Vac_Init="[0,  0,  60]"  Vdc_Init=0  PlotResponse=off  FreqRange=[0, 500, 1]
  Sum : Sum  Inputs=-+  InputSameDT=on  SaturateOnIntegerOverflow=on  OutDataTypeStr=Inherit: Same as first input
  Switch1 : Switch  Criteria=u2 > Threshold
  Switch3 : Switch  Criteria=u2 > Threshold
  Switch4 : Switch  Criteria=u2 > Threshold
  Terminator : Terminator
  Unit Delay : UnitDelay  SampleTime=Ts  HasFrameUpgradeWarning=on
  VR : Fcn  Expr=(u[1] == 2) || (u[1] == 3)
  Voltage Error : Subsystem  TreatAsAtomicUnit=on
  Voltage Regulator : Subsystem  TreatAsAtomicUnit=on
  Voltage dependent Current Order Limiter : Subsystem  mask(Voltage Dependent Current Order Limiter  (Discrete)){Vd_seuil=Vd_seuil, Vd_min=Vd_min, Id_min=Id_min, Id_min_abs=Id_min_abs, Tu=Tup, Ts=Ts}
      mask prompts: Vd_seuil "Vd seuil (pu):"; Vd_min "Vd min (pu):"; Id_min "Id min (pu):"; Id_min_abs "Id min abs (pu):"; Tu "Up Time constant (s):"; Ts "Sample time (s):"
      mask Display: disp('VDCOL\n (Discrete)')
  alpha_init : Subsystem
  alpha_ord (deg) : Outport  VectorParamsAs1DForOutWhenUnconnected=off
  Id_ref_lim : Outport  Port=2  VectorParamsAs1DForOutWhenUnconnected=off
  mode : Outport  Port=3  VectorParamsAs1DForOutWhenUnconnected=off
  wires:
  Voltage Regulator/1(Alpha_ord) -> Switch4/1
  GR/1 -> Gamma Error/Enable, Gamma Regulator/Enable, Switch3/2
  Constant10/1 -> VR/1, GR/1
  VR/1 -> Voltage Error/Enable, Switch4/2, Voltage Regulator/Enable
  D_alpha (deg)/1 -> Alpha Control/2(D_alpha)
  Alpha Control/1(Max_i) -> Current Regulator/1(Max_i), Current Regulator/4(Max_pi), Gamma Regulator/4(Max_pi), Gamma Regulator/1(Max_i), "Control Mode "/5(Max_i), Voltage Regulator/1(Max_i), Voltage Regulator/4(Max_pi)
  Constant6/1 -> Voltage Regulator/8(Min_lin), Gamma Regulator/8(Min_lin), Current Regulator/8(Min_lin)
  Constant4/1 -> Current Error/2
  Id_ref (pu)/1 -> Voltage dependent Current Order Limiter/1(Id_ref (pu))
  Voltage dependent Current Order Limiter/2(Vd_filt) -> Terminator/1
  Voltage dependent Current Order Limiter/1(Id_ref_lim) -> Id_ref_lim/1, Sum/2, Current Error/3
  Second-Order Filter (fn= f0_V)/1 -> Voltage dependent Current Order Limiter/2(Vd (pu)), Voltage Error/2(Vd_meas)
  Min=0 Max = 10/1 -> Second-Order Filter (fn= f0_V)/1
  VdL (pu)/1 -> Min=0 Max = 10/1
  Id (pu)/1 -> First-Order Filter (T = T_I)/1
  First-Order Filter (T = T_I)/1 -> Sum/1, Current Error/1
  Current Error/1 -> Switch1/3
  MinMax/1 -> alpha_init/1(In1)
  Unit Delay/1 -> Voltage Regulator/6(Alpha_lin), Gamma Regulator/6(Alpha_lin), Current Regulator/6(Alpha_lin)
  alpha_init/1(Out1) -> alpha_ord (deg)/1, Unit Delay/1, "Control Mode "/4(alpha_ord)
  Constant5/1 -> Voltage Regulator/7(Max_lin), Gamma Regulator/7(Max_lin), Current Regulator/7(Max_lin)
  Alpha Control/2(Min_i) -> Current Regulator/5(Min_pi), Current Regulator/2(Min_i), Gamma Regulator/5(Min_pi), Gamma Regulator/2(Min_i), "Control Mode "/6(Min_i), Voltage Regulator/2(Min_i), Voltage Regulator/5(Min_pi)
  Block/1 -> Switch1/2, "Control Mode "/7(Block), Gamma Error/3(Block), Voltage Error/3(Block)
  Constant2/1 -> Voltage Regulator/9(Inv), Gamma Regulator/9(Inv), Current Regulator/9(Inv)
  Switch1/1 -> Current Regulator/3(ERR)
  Gamma Regulator/1(Alpha_ord) -> Switch3/1  "Ag"
  Constant8/1 -> Switch3/3
  Constant9/1 -> Switch4/3
  Current Regulator/1(Alpha_ord) -> MinMax/3, "Control Mode "/1("a_ord_i ")  "Ai"
  Switch3/1 -> MinMax/2, "Control Mode "/3(a_ord_g)
  Switch4/1 -> MinMax/1, "Control Mode "/2(a_ord_v)
  Constant1/1 -> Switch1/1
  Gamma Error/1(ERR_G) -> Gamma Regulator/3(ERR)
  gamma_ref (deg)/1 -> Gamma Error/1(G_ref)
  gamma_meas (deg)/1 -> Gamma Error/2(G_meas)
  Sum/1 -> Voltage Error/4(Id_err), Gamma Error/4(Id_err)  "Id_err"
  Vd_ref (pu)/1 -> Voltage Error/1(Vd_ref)
  Voltage Error/1(ERR_V) -> Voltage Regulator/3(ERR)
  "Control Mode "/1(mode) -> mode/1
  Forced_alpha/1 -> Alpha Control/1(Forced_alpha)

== system North_Country_Grid_2024a/Chateauguay HVDC Back-to-Back Converter/Inverter Control and Protection/Inverter Protections ==
  Uabc (pu) : Inport
  Commutation Failure Prevention Control (CFPREV) : Subsystem  mask(Commutation Failure Prevention Control){STATE=on, T_ss=0.64, ab_level=0.1, ab_gain=25, z_level=0.1, z_gain=25, fn=60, Filter=[2.0, 1.0], Ts=Ts}
      mask prompts: STATE "ON State"; T_ss "Simulation Steady_State Time (s):"; ab_level "ab level (pu):"; ab_gain "ab gain (deg/pu):"; z_level "z level (pu):"; z_gain "z gain (deg/pu):"; fn "Base frequency (Hz):"; Filter "Filter Time const. and Iinitial condition [T(s), Ic (pu)]:"; Ts "Sample Time (s):"
      mask help:
      | The protective function, used in the inverter, mitigates commutation failures due to AC voltage dips. After a fault detection (three-phase or one-phase) an angle value (AMIN_CFPREV) is sent to the converter control in order to be deducted from the maximum delay angle limit (alpha_max). Practically, the commutation margin is consequently enlarged reducing therefore the risk of commutation failures.
      |
      |      The CLARK transformation is used for three-phase fault  detection and the zero-sequence voltage evaluation. The detection is based  on instantaneous values, which ensure fast reaction of the control system when AC faults occurs.
      |
      |      Press Help to get the reference with the  detailed description of the function and  parameters.
      |
      | Note: To accelerate the function initialisation, the first parameter (Simulation Steady_State Time) is used. It corresponds to the time when the input voltages reache  the steady-state value.
      mask init:
      | T_periode = 0.6/fn;    % More then half the period
      | filt_tc = Filter(1);
      | filt_ic = Filter(2);
      | 
      | if (STATE)
      | 	str = 'ON';
      | else
      | 	str = 'OFF';
      | end
      mask Help:
      | Ref. "A Novel Method to Mitigate Commutation Failures in HVDC Systems,"
      | Lidong Zhang, Lars Dofnas ABB Utilities Power System Technology,
      | Proceedings PowerCon 2002, Volume: 1 , 13-17 Oct. 2002,  Page(s): 51-56 vol.1.
      mask Display: disp(['\n\n\n State:[',str,']'])
  First-Order Filter (T= 3.3 ms) : spsFirstOrderFilterLib/First-Order Filter  FilterType=Lowpass  Tc=0.0033  Ts=Ts  Initialize=off  Vac_Init=[0, 0, 60]  Vdc_Init=0  PlotResponse=off  FreqRange="[0,  200,  1]"
  Informations : Subsystem
      mask Display: disp('?')
  Low  AC Voltage Detection (LACVD) : Subsystem  TreatAsAtomicUnit=on  mask(Low AC voltage detection){STATE=on, Ref_1=0.75, Ts=fix(0.001/Ts)*Ts}
      mask prompts: STATE "ON State"; Ref_1 "Detection level (pu):"; Ts "Sample time (s):"
      mask help:
      | This bloc detects a low AC voltage condition on the commutation busbar and is used in the DC protection scheme. Its purpose is to descriminate between a drop in the AC voltage caused by a fault on the DC line or by a fault on the AC side.
      |
      |      An AC fault detection (Low_ac_voltage output signal) will occur when the AC voltage input (recified three-phase AC voltage) drops below a certain reference value (Detection level).
      |
      |      In order to minimize the simulation time, an enabled subsystem having a sample time of 1 (ms) has been used in accordance with an acceptable precision.
      mask init:
      | if (STATE)
      | 	str = 'ON';
      | else
      | 	str = 'OFF';
      | end
      mask Display: disp(['\n\n\n\nState:[',str,']'])
  T = 1 ms : DiscretePulseGenerator  Period=fix(0.001/Ts)  SampleTime=Ts
  Udio_6p : Subsystem
  Low_AC_Voltage : Outport  VectorParamsAs1DForOutWhenUnconnected=off
  AMIN_CFPREV : Outport  Port=2  VectorParamsAs1DForOutWhenUnconnected=off
  wires:
  Uabc (pu)/1 -> Udio_6p/1(Uabc (pu)), Commutation Failure Prevention Control (CFPREV)/1(Uabc (pu))
  Low  AC Voltage Detection (LACVD)/1(Low_AC_Voltage) -> Low_AC_Voltage/1
  Commutation Failure Prevention Control (CFPREV)/1(AMIN_CFPREV (deg)) -> AMIN_CFPREV/1
  T = 1 ms/1 -> Low  AC Voltage Detection (LACVD)/Enable
  Udio_6p/1(Udio_6p) -> First-Order Filter (T= 3.3 ms)/1
  First-Order Filter (T= 3.3 ms)/1 -> Low  AC Voltage Detection (LACVD)/1(Uac (pu))

== system North_Country_Grid_2024a/Chateauguay HVDC Back-to-Back Converter/Master Control/Informations ==
  note: For testing purpose,  a step can be activated and added to the reference current at both
      | converters.
  note: Master Control
  note: INTRODUCTION
  note: The rectifier and inverter current reference are generated in the master control. The reference
      | should be equal in both converters to avoid the loss of the margin. The converter starting and stopping is
      | initiated and the current reference can be ramped up or down.  A current step can be added to the
      | current reference for testing purpose.
  note: DESCRIPTION
  note: At start-up, both converters are deblocked and ramped up to the minimum current allowed in steady-state
      | with an adjustable rate  and application time in the "Start/Stop & Ramping Unit" subsystem. After the
      | system stabilisation the current is ramped up to its final value  with an adjustable rate and execution time.
      | Before stopping the converters the current is ramped down to the minimum reference.

== system North_Country_Grid_2024a/Chateauguay HVDC Back-to-Back Converter/Master Control/Start//Stop ==
  note: Start/Stop sequence
  note: Start/Stop & Ramping
  note: Ramping
  Bistable : spsBistableLib/Bistable  Qpriority=Set  ic=0  Ts=Ts
  Edge Detector_1 : spsEdgeDetectorLib/Edge Detector  model=Rising  ic=0  Ts=Ts
  Edge Detector_2 : spsEdgeDetectorLib/Edge Detector  model=Rising  ic=0  Ts=Ts
  Logical Operator3 : Logic  AllPortsSameDT=off
  Minimum ref : Constant  Value=Min_ref
  Relational Operator1 : RelationalOperator  Operator=<=  InputSameDT=off
  S1 : Subsystem  mask(RAMPING UNIT){Min_ref=Min_ref, SS_ramp=SS_ramp, F_up=F_up, up_slope=up_slope, T_up=T_up, F_down=F_down, down_slope=down_slope, T_down=T_down}
      mask prompts: Min_ref "Minimum Value (pu):"; SS_ramp "Start-Stop ramp (pu/s):"; F_up "Final Up Value (pu):"; up_slope "Up Slope (pu/s):"; T_up "Ramping Up Time (s):"; F_down "Final Down Value (pu):"; down_slope "Down Slope (pu/s):"; T_down "Ramping Down Time (s):"
      mask init:
      | T_up_final      =  T_up + (F_up - Min_ref)/up_slope;
      | T_down_final =   T_down + (F_down-F_up)/down_slope;
      | T_ramp  = [0, T_up, T_up_final,  T_down,  T_down_final, 9999]';
      | U_ramp = [0, 0, F_up-Min_ref,  F_up-Min_ref,  F_down- Min_ref,  F_down - Min_ref]';
      mask Display: disp('Ramping\n Unit')
  Start (T_start) : Step  Time=T_start  SampleTime=Ts
  Stop (T_stop) : Step  Time=T_stop  SampleTime=Ts
  Unit Delay : UnitDelay  SampleTime=Ts  HasFrameUpgradeWarning=on
  Id_ref_ramp : Outport  VectorParamsAs1DForOutWhenUnconnected=off
  "Stop " : Outport  Port=2  VectorParamsAs1DForOutWhenUnconnected=off
  wires:
  S1/1(Out1) -> Id_ref_ramp/1
  Minimum ref/1 -> Relational Operator1/2
  Unit Delay/1 -> Relational Operator1/1
  Start (T_start)/1 -> Edge Detector_1/1
  Bistable/1 -> S1/1(Start)  "Start"
  Relational Operator1/1 -> Logical Operator3/1
  Stop (T_stop)/1 -> Logical Operator3/2
  Logical Operator3/1 -> Edge Detector_2/1
  Bistable/2 -> "Stop "/1
  Edge Detector_1/1 -> Bistable/1
  Edge Detector_2/1 -> Bistable/2

== system North_Country_Grid_2024a/Chateauguay HVDC Back-to-Back Converter/Rectifier/Rectifier ==
  Py : Inport
  Pd : Inport  Port=2
  Bridge D : spsUniversalBridgeLib/Universal Bridge  Arms=3  SnubberResistance=2000  SnubberCapacitance=0.1e-6  Device=Thyristors  Ron=1e-3  Lon=0  ForwardVoltages="[  0.8  0.8  ]"  ForwardVoltage=0  GTOparameters=[ 10e-6 , 20e-6 ]  IGBTparameters=[ 1e-6 , 2e-6 ]  Measurements=None  Measurements_2=None  converterType=Rectifier
      settings: AttributesFormatString=\n
  Bridge Y : spsUniversalBridgeLib/Universal Bridge  Arms=3  SnubberResistance=2000  SnubberCapacitance=0.1e-6  Device=Thyristors  Ron=1e-3  Lon=0  ForwardVoltages="[  0.8  0.8  ]"  ForwardVoltage=0  GTOparameters=[ 10e-6 , 20e-6 ]  IGBTparameters=[ 1e-6 , 2e-6 ]  Measurements=All voltages and currents  Measurements_2=None  converterType=Rectifier
      settings: AttributesFormatString=\n
  Ay : PMIOPort  Side=Left
  By : PMIOPort  Port=2  Side=Left
  Cy : PMIOPort  Port=3  Side=Left
  Ad : PMIOPort  Port=4  Side=Left
  Bd : PMIOPort  Port=5  Side=Left
  Cd : PMIOPort  Port=6  Side=Left
  pos : PMIOPort  Port=7  Side=Right
  neg : PMIOPort  Port=8  Side=Right
  wires:
  Pd/1 -> Bridge D/1
  Py/1 -> Bridge Y/1
  connections:
  Bridge D/RConn2 -- neg/RConn1
  Cd/RConn1 -- Bridge D/LConn3
  Bd/RConn1 -- Bridge D/LConn2
  Ad/RConn1 -- Bridge D/LConn1
  Cy/RConn1 -- Bridge Y/LConn3
  By/RConn1 -- Bridge Y/LConn2
  Bridge Y/RConn1 -- pos/RConn1
  Ay/RConn1 -- Bridge Y/LConn1
  Bridge D/RConn1 -- Bridge Y/RConn2
